simulink library "lib_BuildingThermal"  (R2026a)
settings: Solver=VariableStepAuto
libraries: ExternalWall_lib x47, WallSelector_lib x36, RoomWithAirVolume x15, fl_lib x14
(part 1 of 4)
settings Model: Creator=vikrants  LastModifiedBy=vikrants

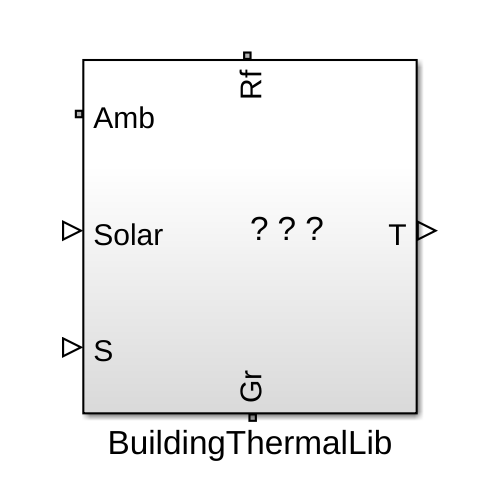
[thumbnail: Simulink's stored preview of the top-level diagram]
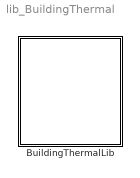
== system lib_BuildingThermal ==
  BuildingThermalLib : Subsystem
      settings: PortSchema="{\"entries\":[{\"content\":{\"sides\":[{\"content\":{\"connectorIds\":[\"LConn1\",\"LConn2\",\"LConn3\"]},\"type\":\"ConnectorPlacement.EquallySpacedRectSide\",\"uuid\":\"02f2e3a8-9f92-46e9-bc8d-cac18fd60cc5\"},{\"content\":{\"connectorIds\":[\"RConn1\"],\"side\":\"RIGHT\"},\"type\":\"ConnectorPlacement.EquallySpacedRectSide\",\"uuid\":\"8e7293df-d9e6-4251-9074-f41050b516bb\"},{\"content\":{\"connectorIds\":[\"LConn4\"],\"side\":\"TOP\"},\"type\":\"ConnectorPlacement.EquallySpacedRectSide\",\"uuid\":\"59004dc2-3d8b-47ae-86a8-cbcf5fc5c8f5\"},{\"content\":{\"connectorIds\":[\"RConn2\"],\"side\":\"BOTTOM\"},\"type\":\"ConnectorPlacement.EquallySpacedRectSide\",\"uuid\":\"040a7ff5-3de3-404c-857a-2e2aad7a1fa3\"}]},\"type\":\"ConnectorPlacement.EquallySpacedConnector\",\"uuid\":\"ad5b2bd3-ca1b-4c9b-b2dc-e1849bcec5d6\"}],\"packageUris\":[\"http://schema.mathworks.com/mf0/Connector/R2020b\"],\"version\":\"1.0\"}"
      mask Display: image('lib_BuildingThermal.png')

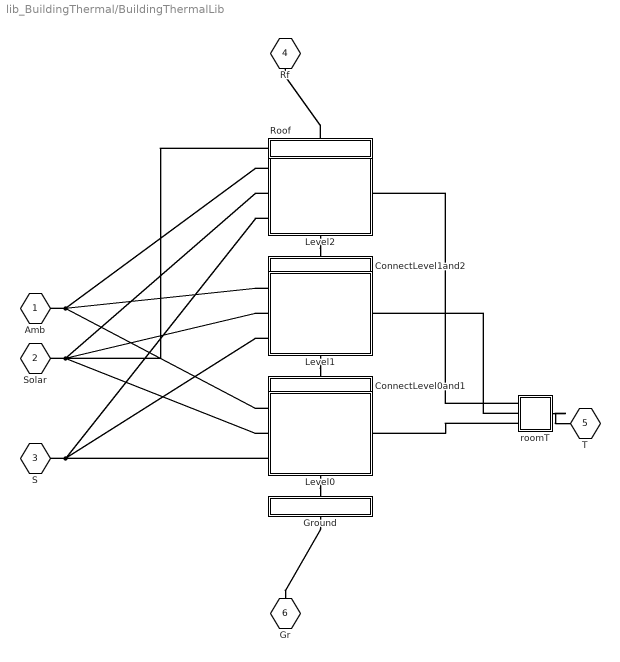
== system lib_BuildingThermal/BuildingThermalLib ==
  ConnectLevel0and1 : Subsystem
      settings: PortSchema="{\"entries\":[{\"content\":{\"sides\":[{\"content\":{},\"type\":\"ConnectorPlacement.EquallySpacedRectSide\",\"uuid\":\"3fb70943-7938-4a07-9cd8-fdf0c154c089\"},{\"content\":{\"side\":\"RIGHT\"},\"type\":\"ConnectorPlacement.EquallySpacedRectSide\",\"uuid\":\"05a521c1-d6a1-4200-9b83-3d3259291215\"},{\"content\":{\"connectorIds\":[\"LConn1\"],\"side\":\"TOP\"},\"type\":\"ConnectorPlacement.EquallySpacedRectSide\",\"uuid\":\"456762b1-d32b-4bbd-9eba-67814e0f7e29\"},{\"content\":{\"connectorIds\":[\"RConn1\"],\"side\":\"BOTTOM\"},\"type\":\"ConnectorPlacement.EquallySpacedRectSide\",\"uuid\":\"1a1553e8-829a-4052-a1db-9258c9d2d2eb\"}]},\"type\":\"ConnectorPlacement.EquallySpacedConnector\",\"uuid\":\"0515c11f-813e-422f-b873-cfb943be20a0\"}],\"packageUris\":[\"http://schema.mathworks.com/mf0/Connector/R2020b\"],\"version\":\"1.0\"}"
  ConnectLevel1and2 : Subsystem
      settings: PortSchema="{\"entries\":[{\"content\":{\"sides\":[{\"content\":{},\"type\":\"ConnectorPlacement.EquallySpacedRectSide\",\"uuid\":\"3fb70943-7938-4a07-9cd8-fdf0c154c089\"},{\"content\":{\"side\":\"RIGHT\"},\"type\":\"ConnectorPlacement.EquallySpacedRectSide\",\"uuid\":\"05a521c1-d6a1-4200-9b83-3d3259291215\"},{\"content\":{\"connectorIds\":[\"LConn1\"],\"side\":\"TOP\"},\"type\":\"ConnectorPlacement.EquallySpacedRectSide\",\"uuid\":\"456762b1-d32b-4bbd-9eba-67814e0f7e29\"},{\"content\":{\"connectorIds\":[\"RConn1\"],\"side\":\"BOTTOM\"},\"type\":\"ConnectorPlacement.EquallySpacedRectSide\",\"uuid\":\"4a30b949-be85-43d7-93f8-e85595850486\"}]},\"type\":\"ConnectorPlacement.EquallySpacedConnector\",\"uuid\":\"0515c11f-813e-422f-b873-cfb943be20a0\"}],\"packageUris\":[\"http://schema.mathworks.com/mf0/Connector/R2020b\"],\"version\":\"1.0\"}"
  Ground : Subsystem
      settings: PortSchema="{\"entries\":[{\"content\":{\"sides\":[{\"content\":{},\"type\":\"ConnectorPlacement.EquallySpacedRectSide\",\"uuid\":\"3fb70943-7938-4a07-9cd8-fdf0c154c089\"},{\"content\":{\"side\":\"RIGHT\"},\"type\":\"ConnectorPlacement.EquallySpacedRectSide\",\"uuid\":\"05a521c1-d6a1-4200-9b83-3d3259291215\"},{\"content\":{\"connectorIds\":[\"LConn1\"],\"side\":\"TOP\"},\"type\":\"ConnectorPlacement.EquallySpacedRectSide\",\"uuid\":\"456762b1-d32b-4bbd-9eba-67814e0f7e29\"},{\"content\":{\"connectorIds\":[\"RConn1\"],\"side\":\"BOTTOM\"},\"type\":\"ConnectorPlacement.EquallySpacedRectSide\",\"uuid\":\"a4d2ba80-0adb-4d34-9370-eb9583c2211d\"}]},\"type\":\"ConnectorPlacement.EquallySpacedConnector\",\"uuid\":\"0515c11f-813e-422f-b873-cfb943be20a0\"}],\"packageUris\":[\"http://schema.mathworks.com/mf0/Connector/R2020b\"],\"version\":\"1.0\"}"
  Level0 : Subsystem
      settings: PortSchema="{\"entries\":[{\"content\":{\"sides\":[{\"content\":{\"connectorIds\":[\"LConn1\",\"LConn2\",\"LConn3\"]},\"type\":\"ConnectorPlacement.EquallySpacedRectSide\",\"uuid\":\"5074afe5-1eb3-4154-99f1-11d56108c9ad\"},{\"content\":{\"connectorIds\":[\"RConn1\"],\"side\":\"RIGHT\"},\"type\":\"ConnectorPlacement.EquallySpacedRectSide\",\"uuid\":\"e70542b5-eb54-43d5-a4ec-335ad714f0fc\"},{\"content\":{\"connectorIds\":[\"LConn4\"],\"side\":\"TOP\"},\"type\":\"ConnectorPlacement.EquallySpacedRectSide\",\"uuid\":\"d6546cf1-a767-41eb-8f4c-4906164cfa57\"},{\"content\":{\"connectorIds\":[\"RConn2\"],\"side\":\"BOTTOM\"},\"type\":\"ConnectorPlacement.EquallySpacedRectSide\",\"uuid\":\"8d7be69c-f27b-4abc-b500-3a84c55d47c4\"}]},\"type\":\"ConnectorPlacement.EquallySpacedConnector\",\"uuid\":\"ebb60fe0-0ae9-4e41-adc3-c2c3cb70ecfc\"}],\"packageUris\":[\"http://schema.mathworks.com/mf0/Connector/R2020b\"],\"version\":\"1.0\"}"
  Level1 : Subsystem
      settings: PortSchema="{\"entries\":[{\"content\":{\"sides\":[{\"content\":{\"connectorIds\":[\"LConn1\",\"LConn2\",\"LConn3\"]},\"type\":\"ConnectorPlacement.EquallySpacedRectSide\",\"uuid\":\"5074afe5-1eb3-4154-99f1-11d56108c9ad\"},{\"content\":{\"connectorIds\":[\"RConn1\"],\"side\":\"RIGHT\"},\"type\":\"ConnectorPlacement.EquallySpacedRectSide\",\"uuid\":\"e70542b5-eb54-43d5-a4ec-335ad714f0fc\"},{\"content\":{\"connectorIds\":[\"LConn4\"],\"side\":\"TOP\"},\"type\":\"ConnectorPlacement.EquallySpacedRectSide\",\"uuid\":\"d6546cf1-a767-41eb-8f4c-4906164cfa57\"},{\"content\":{\"connectorIds\":[\"RConn2\"],\"side\":\"BOTTOM\"},\"type\":\"ConnectorPlacement.EquallySpacedRectSide\",\"uuid\":\"0ce4d1e7-6fe2-4298-a820-c321d652306b\"}]},\"type\":\"ConnectorPlacement.EquallySpacedConnector\",\"uuid\":\"ebb60fe0-0ae9-4e41-adc3-c2c3cb70ecfc\"}],\"packageUris\":[\"http://schema.mathworks.com/mf0/Connector/R2020b\"],\"version\":\"1.0\"}"
  Level2 : Subsystem
      settings: PortSchema="{\"entries\":[{\"content\":{\"sides\":[{\"content\":{\"connectorIds\":[\"LConn1\",\"LConn2\",\"LConn3\"]},\"type\":\"ConnectorPlacement.EquallySpacedRectSide\",\"uuid\":\"5074afe5-1eb3-4154-99f1-11d56108c9ad\"},{\"content\":{\"connectorIds\":[\"RConn1\"],\"side\":\"RIGHT\"},\"type\":\"ConnectorPlacement.EquallySpacedRectSide\",\"uuid\":\"e70542b5-eb54-43d5-a4ec-335ad714f0fc\"},{\"content\":{\"connectorIds\":[\"LConn4\"],\"side\":\"TOP\"},\"type\":\"ConnectorPlacement.EquallySpacedRectSide\",\"uuid\":\"d6546cf1-a767-41eb-8f4c-4906164cfa57\"},{\"content\":{\"connectorIds\":[\"RConn2\"],\"side\":\"BOTTOM\"},\"type\":\"ConnectorPlacement.EquallySpacedRectSide\",\"uuid\":\"ae0b0ecc-8cea-42a6-9f86-a2fcc6949a4a\"}]},\"type\":\"ConnectorPlacement.EquallySpacedConnector\",\"uuid\":\"ebb60fe0-0ae9-4e41-adc3-c2c3cb70ecfc\"}],\"packageUris\":[\"http://schema.mathworks.com/mf0/Connector/R2020b\"],\"version\":\"1.0\"}"
  Roof : Subsystem
      settings: PortSchema="{\"entries\":[{\"content\":{\"sides\":[{\"content\":{\"connectorIds\":[\"LConn1\"]},\"type\":\"ConnectorPlacement.EquallySpacedRectSide\",\"uuid\":\"0be4c07b-4a16-48eb-ba1a-eb19140d6e21\"},{\"content\":{\"side\":\"RIGHT\"},\"type\":\"ConnectorPlacement.EquallySpacedRectSide\",\"uuid\":\"1d83c5b9-3651-480e-b537-4a87f3d8118d\"},{\"content\":{\"connectorIds\":[\"LConn2\"],\"side\":\"TOP\"},\"type\":\"ConnectorPlacement.EquallySpacedRectSide\",\"uuid\":\"3c581fde-8499-4f6e-8539-a668eefd365a\"},{\"content\":{\"connectorIds\":[\"RConn1\"],\"side\":\"BOTTOM\"},\"type\":\"ConnectorPlacement.EquallySpacedRectSide\",\"uuid\":\"56c2556b-374c-4a46-bad4-c741fb2c6272\"}]},\"type\":\"ConnectorPlacement.EquallySpacedConnector\",\"uuid\":\"dfabb703-80b0-43fd-81cb-1196e1f2c066\"}],\"packageUris\":[\"http://schema.mathworks.com/mf0/Connector/R2020b\"],\"version\":\"1.0\"}"
  roomT : Subsystem
  Amb : PMIOPort  Side=Left
  Solar : PMIOPort  Port=2  Side=Left
  S : PMIOPort  Port=3  Side=Left
  Rf : PMIOPort  Port=4  Side=Left
  T : PMIOPort  Port=5  Side=Right
  Gr : PMIOPort  Port=6  Side=Right
  connections:
  Level0/RConn2 -- Ground/LConn1
  Level1/RConn2 -- ConnectLevel0and1/LConn1
  Level0/LConn4 -- ConnectLevel0and1/RConn1
  Level2/RConn2 -- ConnectLevel1and2/LConn1
  Level1/LConn4 -- ConnectLevel1and2/RConn1
  Level2/LConn4 -- Roof/RConn1
  Roof/LConn2 -- Rf/RConn1
  Ground/RConn1 -- Gr/RConn1
  Roof/LConn1 -- Level0/LConn2 -- Level1/LConn2 -- Solar/RConn1 -- Level2/LConn2
  Level0/LConn1 -- Level1/LConn1 -- Amb/RConn1 -- Level2/LConn1
  Level0/LConn3 -- Level1/LConn3 -- S/RConn1 -- Level2/LConn3
  roomT/LConn1 -- Level2/RConn1
  roomT/LConn2 -- Level1/RConn1
  roomT/LConn3 -- Level0/RConn1
  roomT/RConn1 -- T/RConn1

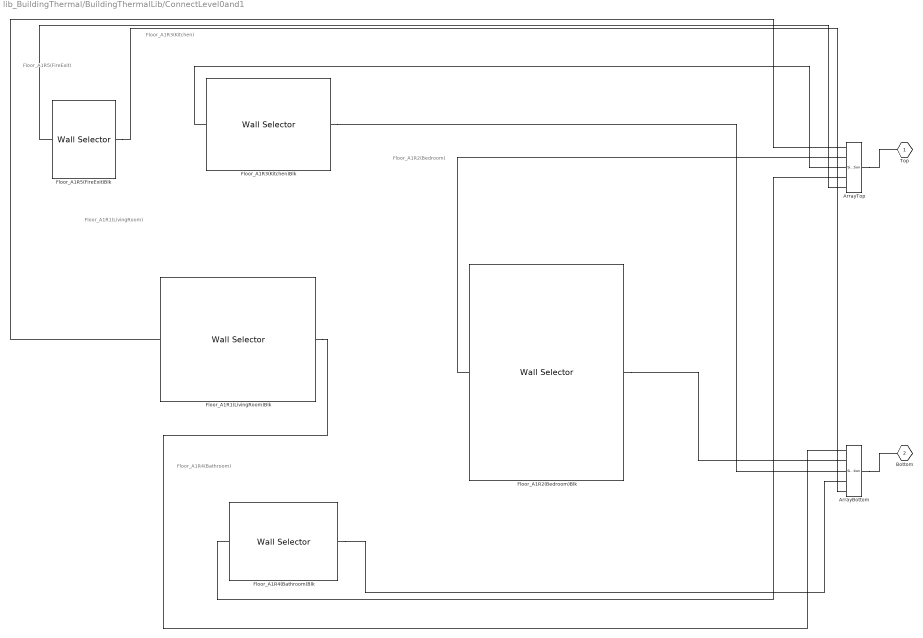
== system lib_BuildingThermal/BuildingThermalLib/ConnectLevel0and1 ==
  note: Floor_A1R1(LivingRoom)
  note: Floor_A1R2(Bedroom)
  note: Floor_A1R3(Kitchen)
  note: Floor_A1R4(Bathroom)
  note: Floor_A1R5(FireExit)
  ArrayBottom : SimscapeArrayConnection  Domain=foundation.thermal.thermal  ConcatenateDimension=1  NumScalarElements=5
  ArrayTop : SimscapeArrayConnection  Domain=foundation.thermal.thermal  ConcatenateDimension=1  NumScalarElements=5
  Floor_A1R1(LivingRoom)Blk : WallSelector_lib/Wall Selector  optWall=wallModelOption.wallOnly  wallLength=2.4384 % Parameterized on : 09-Jun-2026 19:35:13 m  wallHeight=3.048 % Parameterized on : 09-Jun-2026 19:35:13 m  wallThickness=0.03 % Parameterized on : 09-Jun-2026 19:35:13 m  wallMaterialDen=1400 % Parameterized on : 09-Jun-2026 19:35:15 kg/m^3  wallMaterialCp=1000 % Parameterized on : 09-Jun-2026 19:35:15 J/(K*kg)  wallAbsorptivity=0.5  wallThermalK=0.7 % Parameterized on : 09-Jun-2026 19:35:15 W/(K*m)  winLength=1 m  winHeight=0.5 m  winThickness=0.007 m  winMaterialDen=2500 kg/m^3  winMaterialCp=787 J/(K*kg)  winAbsorptivity=0.35  winThermalK=1 W/(K*m)  winTransmissivity=0.45  ventLength=0.1 m  ventHeight=0.1 m  extToWallHTC=30 % Parameterized on : 09-Jun-2026 19:35:15 W/(K*m^2)  intToRoomHTC=30 % Parameterized on : 09-Jun-2026 19:35:15 W/(K*m^2)  iniT=300 % Parameterized on : 09-Jun-2026 19:35:15 K
  Floor_A1R2(Bedroom)Blk : WallSelector_lib/Wall Selector  optWall=wallModelOption.wallOnly  wallLength=4.2672 % Parameterized on : 09-Jun-2026 19:35:13 m  wallHeight=3.048 % Parameterized on : 09-Jun-2026 19:35:13 m  wallThickness=0.03 % Parameterized on : 09-Jun-2026 19:35:13 m  wallMaterialDen=1400 % Parameterized on : 09-Jun-2026 19:35:15 kg/m^3  wallMaterialCp=1000 % Parameterized on : 09-Jun-2026 19:35:15 J/(K*kg)  wallAbsorptivity=0.5  wallThermalK=0.7 % Parameterized on : 09-Jun-2026 19:35:15 W/(K*m)  winLength=1 m  winHeight=0.5 m  winThickness=0.007 m  winMaterialDen=2500 kg/m^3  winMaterialCp=787 J/(K*kg)  winAbsorptivity=0.35  winThermalK=1 W/(K*m)  winTransmissivity=0.45  ventLength=0.1 m  ventHeight=0.1 m  extToWallHTC=30 % Parameterized on : 09-Jun-2026 19:35:15 W/(K*m^2)  intToRoomHTC=30 % Parameterized on : 09-Jun-2026 19:35:15 W/(K*m^2)  iniT=300 % Parameterized on : 09-Jun-2026 19:35:15 K
  Floor_A1R3(Kitchen)Blk : WallSelector_lib/Wall Selector  optWall=wallModelOption.wallOnly  wallLength=1.8288 % Parameterized on : 09-Jun-2026 19:35:13 m  wallHeight=2.4384 % Parameterized on : 09-Jun-2026 19:35:13 m  wallThickness=0.03 % Parameterized on : 09-Jun-2026 19:35:13 m  wallMaterialDen=1400 % Parameterized on : 09-Jun-2026 19:35:15 kg/m^3  wallMaterialCp=1000 % Parameterized on : 09-Jun-2026 19:35:15 J/(K*kg)  wallAbsorptivity=0.5  wallThermalK=0.7 % Parameterized on : 09-Jun-2026 19:35:15 W/(K*m)  winLength=1 m  winHeight=0.5 m  winThickness=0.007 m  winMaterialDen=2500 kg/m^3  winMaterialCp=787 J/(K*kg)  winAbsorptivity=0.35  winThermalK=1 W/(K*m)  winTransmissivity=0.45  ventLength=0.1 m  ventHeight=0.1 m  extToWallHTC=30 % Parameterized on : 09-Jun-2026 19:35:15 W/(K*m^2)  intToRoomHTC=30 % Parameterized on : 09-Jun-2026 19:35:15 W/(K*m^2)  iniT=300 % Parameterized on : 09-Jun-2026 19:35:15 K
  Floor_A1R4(Bathroom)Blk : WallSelector_lib/Wall Selector  optWall=wallModelOption.wallOnly  wallLength=1.524 % Parameterized on : 09-Jun-2026 19:35:13 m  wallHeight=2.1336 % Parameterized on : 09-Jun-2026 19:35:13 m  wallThickness=0.03 % Parameterized on : 09-Jun-2026 19:35:13 m  wallMaterialDen=1400 % Parameterized on : 09-Jun-2026 19:35:15 kg/m^3  wallMaterialCp=1000 % Parameterized on : 09-Jun-2026 19:35:15 J/(K*kg)  wallAbsorptivity=0.5  wallThermalK=0.7 % Parameterized on : 09-Jun-2026 19:35:15 W/(K*m)  winLength=1 m  winHeight=0.5 m  winThickness=0.007 m  winMaterialDen=2500 kg/m^3  winMaterialCp=787 J/(K*kg)  winAbsorptivity=0.35  winThermalK=1 W/(K*m)  winTransmissivity=0.45  ventLength=0.1 m  ventHeight=0.1 m  extToWallHTC=30 % Parameterized on : 09-Jun-2026 19:35:15 W/(K*m^2)  intToRoomHTC=30 % Parameterized on : 09-Jun-2026 19:35:15 W/(K*m^2)  iniT=300 % Parameterized on : 09-Jun-2026 19:35:15 K
  Floor_A1R5(FireExit)Blk : WallSelector_lib/Wall Selector  optWall=wallModelOption.wallOnly  wallLength=1.524 % Parameterized on : 09-Jun-2026 19:35:13 m  wallHeight=1.2192 % Parameterized on : 09-Jun-2026 19:35:13 m  wallThickness=0.03 % Parameterized on : 09-Jun-2026 19:35:13 m  wallMaterialDen=1400 % Parameterized on : 09-Jun-2026 19:35:15 kg/m^3  wallMaterialCp=1000 % Parameterized on : 09-Jun-2026 19:35:15 J/(K*kg)  wallAbsorptivity=0.5  wallThermalK=0.7 % Parameterized on : 09-Jun-2026 19:35:15 W/(K*m)  winLength=1 m  winHeight=0.5 m  winThickness=0.007 m  winMaterialDen=2500 kg/m^3  winMaterialCp=787 J/(K*kg)  winAbsorptivity=0.35  winThermalK=1 W/(K*m)  winTransmissivity=0.45  ventLength=0.1 m  ventHeight=0.1 m  extToWallHTC=30 % Parameterized on : 09-Jun-2026 19:35:15 W/(K*m^2)  intToRoomHTC=30 % Parameterized on : 09-Jun-2026 19:35:15 W/(K*m^2)  iniT=300 % Parameterized on : 09-Jun-2026 19:35:15 K
  Top : PMIOPort  Side=Left
  Bottom : PMIOPort  Port=2  Side=Right
  connections:
  ArrayTop/RConn1 -- Top/RConn1
  Floor_A1R1(LivingRoom)Blk/LConn1 -- ArrayTop/LConn1
  Floor_A1R2(Bedroom)Blk/LConn1 -- ArrayTop/LConn2
  Floor_A1R3(Kitchen)Blk/LConn1 -- ArrayTop/LConn3
  Floor_A1R4(Bathroom)Blk/LConn1 -- ArrayTop/LConn4
  Floor_A1R5(FireExit)Blk/LConn1 -- ArrayTop/LConn5
  ArrayBottom/RConn1 -- Bottom/RConn1
  Floor_A1R1(LivingRoom)Blk/RConn1 -- ArrayBottom/LConn1
  Floor_A1R2(Bedroom)Blk/RConn1 -- ArrayBottom/LConn2
  Floor_A1R3(Kitchen)Blk/RConn1 -- ArrayBottom/LConn3
  Floor_A1R4(Bathroom)Blk/RConn1 -- ArrayBottom/LConn4
  Floor_A1R5(FireExit)Blk/RConn1 -- ArrayBottom/LConn5

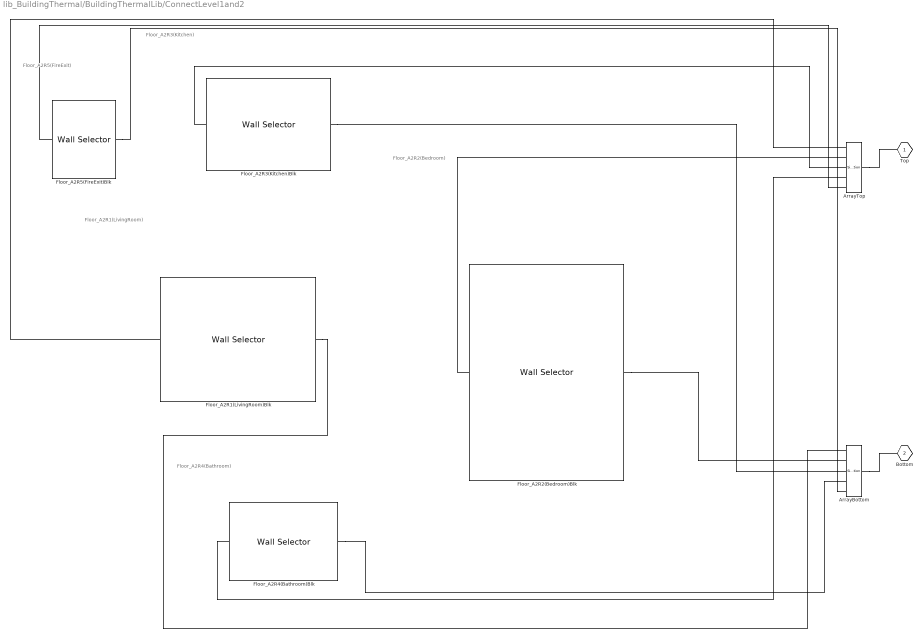
== system lib_BuildingThermal/BuildingThermalLib/ConnectLevel1and2 ==
  note: Floor_A2R1(LivingRoom)
  note: Floor_A2R2(Bedroom)
  note: Floor_A2R3(Kitchen)
  note: Floor_A2R4(Bathroom)
  note: Floor_A2R5(FireExit)
  ArrayBottom : SimscapeArrayConnection  Domain=foundation.thermal.thermal  ConcatenateDimension=1  NumScalarElements=5
  ArrayTop : SimscapeArrayConnection  Domain=foundation.thermal.thermal  ConcatenateDimension=1  NumScalarElements=5
  Floor_A2R1(LivingRoom)Blk : WallSelector_lib/Wall Selector  optWall=wallModelOption.wallOnly  wallLength=2.4384 % Parameterized on : 09-Jun-2026 19:35:13 m  wallHeight=3.048 % Parameterized on : 09-Jun-2026 19:35:13 m  wallThickness=0.03 % Parameterized on : 09-Jun-2026 19:35:13 m  wallMaterialDen=1400 % Parameterized on : 09-Jun-2026 19:35:15 kg/m^3  wallMaterialCp=1000 % Parameterized on : 09-Jun-2026 19:35:15 J/(K*kg)  wallAbsorptivity=0.5  wallThermalK=0.7 % Parameterized on : 09-Jun-2026 19:35:15 W/(K*m)  winLength=1 m  winHeight=0.5 m  winThickness=0.007 m  winMaterialDen=2500 kg/m^3  winMaterialCp=787 J/(K*kg)  winAbsorptivity=0.35  winThermalK=1 W/(K*m)  winTransmissivity=0.45  ventLength=0.1 m  ventHeight=0.1 m  extToWallHTC=30 % Parameterized on : 09-Jun-2026 19:35:15 W/(K*m^2)  intToRoomHTC=30 % Parameterized on : 09-Jun-2026 19:35:15 W/(K*m^2)  iniT=300 % Parameterized on : 09-Jun-2026 19:35:15 K
  Floor_A2R2(Bedroom)Blk : WallSelector_lib/Wall Selector  optWall=wallModelOption.wallOnly  wallLength=4.2672 % Parameterized on : 09-Jun-2026 19:35:13 m  wallHeight=3.048 % Parameterized on : 09-Jun-2026 19:35:13 m  wallThickness=0.03 % Parameterized on : 09-Jun-2026 19:35:13 m  wallMaterialDen=1400 % Parameterized on : 09-Jun-2026 19:35:15 kg/m^3  wallMaterialCp=1000 % Parameterized on : 09-Jun-2026 19:35:15 J/(K*kg)  wallAbsorptivity=0.5  wallThermalK=0.7 % Parameterized on : 09-Jun-2026 19:35:15 W/(K*m)  winLength=1 m  winHeight=0.5 m  winThickness=0.007 m  winMaterialDen=2500 kg/m^3  winMaterialCp=787 J/(K*kg)  winAbsorptivity=0.35  winThermalK=1 W/(K*m)  winTransmissivity=0.45  ventLength=0.1 m  ventHeight=0.1 m  extToWallHTC=30 % Parameterized on : 09-Jun-2026 19:35:15 W/(K*m^2)  intToRoomHTC=30 % Parameterized on : 09-Jun-2026 19:35:15 W/(K*m^2)  iniT=300 % Parameterized on : 09-Jun-2026 19:35:15 K
  Floor_A2R3(Kitchen)Blk : WallSelector_lib/Wall Selector  optWall=wallModelOption.wallOnly  wallLength=1.8288 % Parameterized on : 09-Jun-2026 19:35:13 m  wallHeight=2.4384 % Parameterized on : 09-Jun-2026 19:35:13 m  wallThickness=0.03 % Parameterized on : 09-Jun-2026 19:35:13 m  wallMaterialDen=1400 % Parameterized on : 09-Jun-2026 19:35:15 kg/m^3  wallMaterialCp=1000 % Parameterized on : 09-Jun-2026 19:35:15 J/(K*kg)  wallAbsorptivity=0.5  wallThermalK=0.7 % Parameterized on : 09-Jun-2026 19:35:15 W/(K*m)  winLength=1 m  winHeight=0.5 m  winThickness=0.007 m  winMaterialDen=2500 kg/m^3  winMaterialCp=787 J/(K*kg)  winAbsorptivity=0.35  winThermalK=1 W/(K*m)  winTransmissivity=0.45  ventLength=0.1 m  ventHeight=0.1 m  extToWallHTC=30 % Parameterized on : 09-Jun-2026 19:35:15 W/(K*m^2)  intToRoomHTC=30 % Parameterized on : 09-Jun-2026 19:35:15 W/(K*m^2)  iniT=300 % Parameterized on : 09-Jun-2026 19:35:15 K
  Floor_A2R4(Bathroom)Blk : WallSelector_lib/Wall Selector  optWall=wallModelOption.wallOnly  wallLength=1.524 % Parameterized on : 09-Jun-2026 19:35:13 m  wallHeight=2.1336 % Parameterized on : 09-Jun-2026 19:35:13 m  wallThickness=0.03 % Parameterized on : 09-Jun-2026 19:35:13 m  wallMaterialDen=1400 % Parameterized on : 09-Jun-2026 19:35:15 kg/m^3  wallMaterialCp=1000 % Parameterized on : 09-Jun-2026 19:35:15 J/(K*kg)  wallAbsorptivity=0.5  wallThermalK=0.7 % Parameterized on : 09-Jun-2026 19:35:15 W/(K*m)  winLength=1 m  winHeight=0.5 m  winThickness=0.007 m  winMaterialDen=2500 kg/m^3  winMaterialCp=787 J/(K*kg)  winAbsorptivity=0.35  winThermalK=1 W/(K*m)  winTransmissivity=0.45  ventLength=0.1 m  ventHeight=0.1 m  extToWallHTC=30 % Parameterized on : 09-Jun-2026 19:35:15 W/(K*m^2)  intToRoomHTC=30 % Parameterized on : 09-Jun-2026 19:35:15 W/(K*m^2)  iniT=300 % Parameterized on : 09-Jun-2026 19:35:15 K
  Floor_A2R5(FireExit)Blk : WallSelector_lib/Wall Selector  optWall=wallModelOption.wallOnly  wallLength=1.524 % Parameterized on : 09-Jun-2026 19:35:13 m  wallHeight=1.2192 % Parameterized on : 09-Jun-2026 19:35:13 m  wallThickness=0.03 % Parameterized on : 09-Jun-2026 19:35:13 m  wallMaterialDen=1400 % Parameterized on : 09-Jun-2026 19:35:15 kg/m^3  wallMaterialCp=1000 % Parameterized on : 09-Jun-2026 19:35:15 J/(K*kg)  wallAbsorptivity=0.5  wallThermalK=0.7 % Parameterized on : 09-Jun-2026 19:35:15 W/(K*m)  winLength=1 m  winHeight=0.5 m  winThickness=0.007 m  winMaterialDen=2500 kg/m^3  winMaterialCp=787 J/(K*kg)  winAbsorptivity=0.35  winThermalK=1 W/(K*m)  winTransmissivity=0.45  ventLength=0.1 m  ventHeight=0.1 m  extToWallHTC=30 % Parameterized on : 09-Jun-2026 19:35:15 W/(K*m^2)  intToRoomHTC=30 % Parameterized on : 09-Jun-2026 19:35:15 W/(K*m^2)  iniT=300 % Parameterized on : 09-Jun-2026 19:35:15 K
  Top : PMIOPort  Side=Left
  Bottom : PMIOPort  Port=2  Side=Right
  connections:
  ArrayTop/RConn1 -- Top/RConn1
  Floor_A2R1(LivingRoom)Blk/LConn1 -- ArrayTop/LConn1
  Floor_A2R2(Bedroom)Blk/LConn1 -- ArrayTop/LConn2
  Floor_A2R3(Kitchen)Blk/LConn1 -- ArrayTop/LConn3
  Floor_A2R4(Bathroom)Blk/LConn1 -- ArrayTop/LConn4
  Floor_A2R5(FireExit)Blk/LConn1 -- ArrayTop/LConn5
  ArrayBottom/RConn1 -- Bottom/RConn1
  Floor_A2R1(LivingRoom)Blk/RConn1 -- ArrayBottom/LConn1
  Floor_A2R2(Bedroom)Blk/RConn1 -- ArrayBottom/LConn2
  Floor_A2R3(Kitchen)Blk/RConn1 -- ArrayBottom/LConn3
  Floor_A2R4(Bathroom)Blk/RConn1 -- ArrayBottom/LConn4
  Floor_A2R5(FireExit)Blk/RConn1 -- ArrayBottom/LConn5

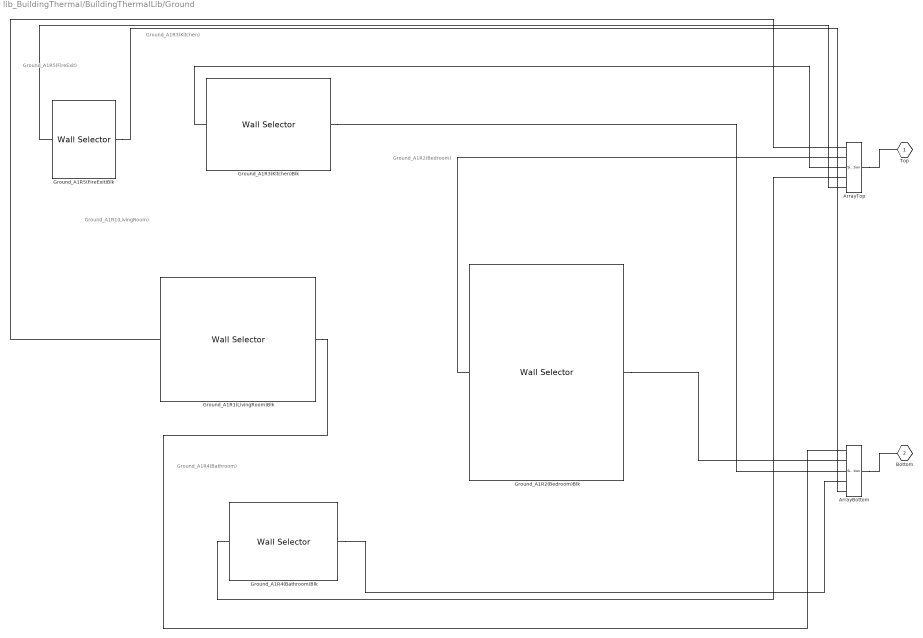
== system lib_BuildingThermal/BuildingThermalLib/Ground ==
  note: Ground_A1R1(LivingRoom)
  note: Ground_A1R2(Bedroom)
  note: Ground_A1R3(Kitchen)
  note: Ground_A1R4(Bathroom)
  note: Ground_A1R5(FireExit)
  ArrayBottom : SimscapeArrayConnection  Domain=foundation.thermal.thermal  ConcatenateDimension=1  NumScalarElements=5
  ArrayTop : SimscapeArrayConnection  Domain=foundation.thermal.thermal  ConcatenateDimension=1  NumScalarElements=5
  Ground_A1R1(LivingRoom)Blk : WallSelector_lib/Wall Selector  optWall=wallModelOption.wallOnly  wallLength=2.4384 % Parameterized on : 09-Jun-2026 19:35:13 m  wallHeight=3.048 % Parameterized on : 09-Jun-2026 19:35:13 m  wallThickness=0.03 % Parameterized on : 09-Jun-2026 19:35:13 m  wallMaterialDen=1400 % Parameterized on : 09-Jun-2026 19:35:15 kg/m^3  wallMaterialCp=1000 % Parameterized on : 09-Jun-2026 19:35:15 J/(K*kg)  wallAbsorptivity=0.5  wallThermalK=0.7 % Parameterized on : 09-Jun-2026 19:35:15 W/(K*m)  winLength=1 m  winHeight=0.5 m  winThickness=0.007 m  winMaterialDen=2500 kg/m^3  winMaterialCp=787 J/(K*kg)  winAbsorptivity=0.35  winThermalK=1 W/(K*m)  winTransmissivity=0.45  ventLength=0.1 m  ventHeight=0.1 m  extToWallHTC=30 % Parameterized on : 09-Jun-2026 19:35:15 W/(K*m^2)  intToRoomHTC=30 % Parameterized on : 09-Jun-2026 19:35:15 W/(K*m^2)  iniT=300 % Parameterized on : 09-Jun-2026 19:35:15 K
  Ground_A1R2(Bedroom)Blk : WallSelector_lib/Wall Selector  optWall=wallModelOption.wallOnly  wallLength=4.2672 % Parameterized on : 09-Jun-2026 19:35:13 m  wallHeight=3.048 % Parameterized on : 09-Jun-2026 19:35:13 m  wallThickness=0.03 % Parameterized on : 09-Jun-2026 19:35:13 m  wallMaterialDen=1400 % Parameterized on : 09-Jun-2026 19:35:15 kg/m^3  wallMaterialCp=1000 % Parameterized on : 09-Jun-2026 19:35:15 J/(K*kg)  wallAbsorptivity=0.5  wallThermalK=0.7 % Parameterized on : 09-Jun-2026 19:35:16 W/(K*m)  winLength=1 m  winHeight=0.5 m  winThickness=0.007 m  winMaterialDen=2500 kg/m^3  winMaterialCp=787 J/(K*kg)  winAbsorptivity=0.35  winThermalK=1 W/(K*m)  winTransmissivity=0.45  ventLength=0.1 m  ventHeight=0.1 m  extToWallHTC=30 % Parameterized on : 09-Jun-2026 19:35:16 W/(K*m^2)  intToRoomHTC=30 % Parameterized on : 09-Jun-2026 19:35:16 W/(K*m^2)  iniT=300 % Parameterized on : 09-Jun-2026 19:35:16 K
  Ground_A1R3(Kitchen)Blk : WallSelector_lib/Wall Selector  optWall=wallModelOption.wallOnly  wallLength=1.8288 % Parameterized on : 09-Jun-2026 19:35:13 m  wallHeight=2.4384 % Parameterized on : 09-Jun-2026 19:35:13 m  wallThickness=0.03 % Parameterized on : 09-Jun-2026 19:35:13 m  wallMaterialDen=1400 % Parameterized on : 09-Jun-2026 19:35:16 kg/m^3  wallMaterialCp=1000 % Parameterized on : 09-Jun-2026 19:35:16 J/(K*kg)  wallAbsorptivity=0.5  wallThermalK=0.7 % Parameterized on : 09-Jun-2026 19:35:16 W/(K*m)  winLength=1 m  winHeight=0.5 m  winThickness=0.007 m  winMaterialDen=2500 kg/m^3  winMaterialCp=787 J/(K*kg)  winAbsorptivity=0.35  winThermalK=1 W/(K*m)  winTransmissivity=0.45  ventLength=0.1 m  ventHeight=0.1 m  extToWallHTC=30 % Parameterized on : 09-Jun-2026 19:35:16 W/(K*m^2)  intToRoomHTC=30 % Parameterized on : 09-Jun-2026 19:35:16 W/(K*m^2)  iniT=300 % Parameterized on : 09-Jun-2026 19:35:16 K
  Ground_A1R4(Bathroom)Blk : WallSelector_lib/Wall Selector  optWall=wallModelOption.wallOnly  wallLength=1.524 % Parameterized on : 09-Jun-2026 19:35:13 m  wallHeight=2.1336 % Parameterized on : 09-Jun-2026 19:35:13 m  wallThickness=0.03 % Parameterized on : 09-Jun-2026 19:35:13 m  wallMaterialDen=1400 % Parameterized on : 09-Jun-2026 19:35:16 kg/m^3  wallMaterialCp=1000 % Parameterized on : 09-Jun-2026 19:35:16 J/(K*kg)  wallAbsorptivity=0.5  wallThermalK=0.7 % Parameterized on : 09-Jun-2026 19:35:16 W/(K*m)  winLength=1 m  winHeight=0.5 m  winThickness=0.007 m  winMaterialDen=2500 kg/m^3  winMaterialCp=787 J/(K*kg)  winAbsorptivity=0.35  winThermalK=1 W/(K*m)  winTransmissivity=0.45  ventLength=0.1 m  ventHeight=0.1 m  extToWallHTC=30 % Parameterized on : 09-Jun-2026 19:35:16 W/(K*m^2)  intToRoomHTC=30 % Parameterized on : 09-Jun-2026 19:35:16 W/(K*m^2)  iniT=300 % Parameterized on : 09-Jun-2026 19:35:16 K
  Ground_A1R5(FireExit)Blk : WallSelector_lib/Wall Selector  optWall=wallModelOption.wallOnly  wallLength=1.524 % Parameterized on : 09-Jun-2026 19:35:13 m  wallHeight=1.2192 % Parameterized on : 09-Jun-2026 19:35:13 m  wallThickness=0.03 % Parameterized on : 09-Jun-2026 19:35:13 m  wallMaterialDen=1400 % Parameterized on : 09-Jun-2026 19:35:16 kg/m^3  wallMaterialCp=1000 % Parameterized on : 09-Jun-2026 19:35:16 J/(K*kg)  wallAbsorptivity=0.5  wallThermalK=0.7 % Parameterized on : 09-Jun-2026 19:35:16 W/(K*m)  winLength=1 m  winHeight=0.5 m  winThickness=0.007 m  winMaterialDen=2500 kg/m^3  winMaterialCp=787 J/(K*kg)  winAbsorptivity=0.35  winThermalK=1 W/(K*m)  winTransmissivity=0.45  ventLength=0.1 m  ventHeight=0.1 m  extToWallHTC=30 % Parameterized on : 09-Jun-2026 19:35:16 W/(K*m^2)  intToRoomHTC=30 % Parameterized on : 09-Jun-2026 19:35:16 W/(K*m^2)  iniT=300 % Parameterized on : 09-Jun-2026 19:35:16 K
  Top : PMIOPort  Side=Left
  Bottom : PMIOPort  Port=2  Side=Right
  connections:
  ArrayTop/RConn1 -- Top/RConn1
  Ground_A1R1(LivingRoom)Blk/LConn1 -- ArrayTop/LConn1
  Ground_A1R2(Bedroom)Blk/LConn1 -- ArrayTop/LConn2
  Ground_A1R3(Kitchen)Blk/LConn1 -- ArrayTop/LConn3
  Ground_A1R4(Bathroom)Blk/LConn1 -- ArrayTop/LConn4
  Ground_A1R5(FireExit)Blk/LConn1 -- ArrayTop/LConn5
  ArrayBottom/RConn1 -- Bottom/RConn1
  Ground_A1R1(LivingRoom)Blk/RConn1 -- ArrayBottom/LConn1
  Ground_A1R2(Bedroom)Blk/RConn1 -- ArrayBottom/LConn2
  Ground_A1R3(Kitchen)Blk/RConn1 -- ArrayBottom/LConn3
  Ground_A1R4(Bathroom)Blk/RConn1 -- ArrayBottom/LConn4
  Ground_A1R5(FireExit)Blk/RConn1 -- ArrayBottom/LConn5
